simulink subsystem "Eulers_Equation"  (R2023b)
settings: Solver=VariableStepAuto  StartTime=0.0  StopTime=10.0  RelTol=1e-3
libraries: matrix_library x1, aerolibutil x1
settings Model: Creator=Andrew Radulovich  LastModifiedBy=thatf
settings ModelReferenceCC: EnableRefExpFcnMdlSchedulingChecks=on

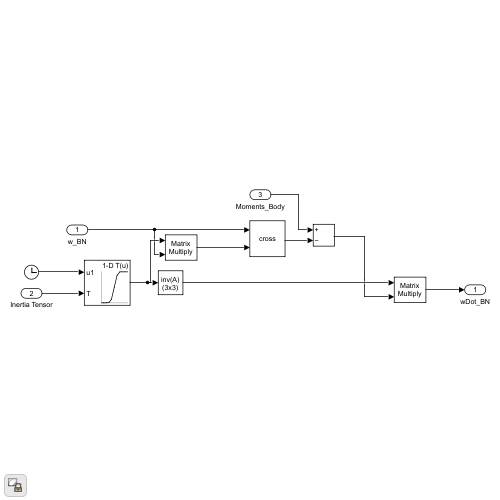
[thumbnail: Simulink's stored preview of the top-level diagram]
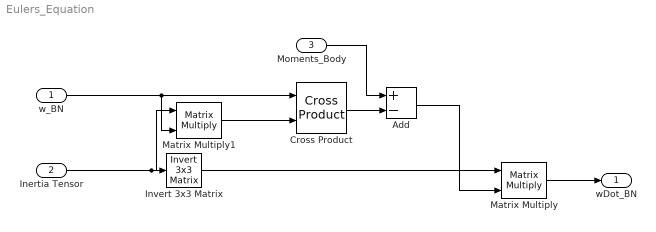
== system Eulers_Equation ==
  w_BN : Inport
  Inertia Tensor : Inport  Port=2
  Moments_Body : Inport  Port=3
  Add : Sum  Inputs=+-
  Cross Product : matrix_library/Cross Product
  Invert 3x3 Matrix : aerolibutil/Invert  3x3 Matrix
  Matrix Multiply : Product  Multiplication=Matrix(*)
  Matrix Multiply1 : Product  Multiplication=Matrix(*)
  wDot_BN : Outport
  wires:
  Inertia Tensor/1 -> Matrix Multiply1/1, Invert 3x3 Matrix/1
  Matrix Multiply/1 -> wDot_BN/1
  Add/1 -> Matrix Multiply/2
  Moments_Body/1 -> Add/1
  Cross Product/1 -> Add/2
  Matrix Multiply1/1 -> Cross Product/2
  w_BN/1 -> Matrix Multiply1/2, Cross Product/1
  Invert 3x3 Matrix/1 -> Matrix Multiply/1
